simulink model "CF010A_GmTqArbn"  (R2013b)
settings: Solver=FixedStepDiscrete  SolverMode=SingleTasking  StartTime=0.0  StopTime=1  FixedStep=0.002  RelTol=1e-3
values from neighbouring files (symbols this model uses):
  ARCHGLBPRM_2MILLISEC_SEC_F32 = DataDict.Constant    [CF010A_GmTqArbn_DataDict.m]
  ESCTQCMDOVRLLIM_HWNWTMTR_F32 = DataDict.Constant    [CF010A_GmTqArbn_DataDict.m]
  FINALSLEWLWRLIM_HWNWTMTRPERSEC_F32 = DataDict.Constant    [CF010A_GmTqArbn_DataDict.m]
  GmTqArbnApaAssiScaEna = DataDict.Calibration    [CF010A_GmTqArbn_DataDict.m]
  GmTqArbnApaDampgScaEna = DataDict.Calibration    [CF010A_GmTqArbn_DataDict.m]
  GmTqArbnApaEnaRate = DataDict.Calibration    [CF010A_GmTqArbn_DataDict.m]
  GmTqArbnApaRtnScaEna = DataDict.Calibration    [CF010A_GmTqArbn_DataDict.m]
  GmTqArbnEscMaxTq = DataDict.Calibration    [CF010A_GmTqArbn_DataDict.m]
  GmTqArbnLkaOutpOvrlUpprLim = DataDict.Calibration    [CF010A_GmTqArbn_DataDict.m]
  GmTqArbnLkaSlewEna = DataDict.Calibration    [CF010A_GmTqArbn_DataDict.m]
  HWTQCMDOVRLLIM_HWNWTMTR_F32 = DataDict.Constant    [CF010A_GmTqArbn_DataDict.m]
  LKACMDHILIM_HWNWTMTR_F32 = DataDict.Constant    [CF010A_GmTqArbn_DataDict.m]
  LKAOUTPOVRLLIM_MOTNWTMTR_F32 = DataDict.Constant    [CF010A_GmTqArbn_DataDict.m]
  LKATQCMDOVRLLIM_HWNWTMTR_F32 = DataDict.Constant    [CF010A_GmTqArbn_DataDict.m]
  MOTTQCMDOVRLLIM_MOTNWTMTR_F32 = DataDict.Constant    [CF010A_GmTqArbn_DataDict.m]
  OUTPCMDHILIM_ULS_F32 = DataDict.Constant    [CF010A_GmTqArbn_DataDict.m]
  OUTPCMDLOWRLIM_ULS_F32 = DataDict.Constant    [CF010A_GmTqArbn_DataDict.m]
  POSNSERVOSMOOTHMINLWRLIM_ULSPERSEC_F32 = DataDict.Constant    [CF010A_GmTqArbn_DataDict.m]
  VELDPTTQOVRLMTRCOFFS_HWNWTMTRPERSEC_F32 = DataDict.Constant    [CF010A_GmTqArbn_DataDict.m]
  VELDPTTQOVRLMTRCTQPERVEHSPD_HWNWTMTRPERSECPERKPH_F32 = DataDict.Constant    [CF010A_GmTqArbn_DataDict.m]
undefined symbols (not defined in the file or in its folder): GmTqArbnEscSt1, GmTqArbnLkaSt1
libraries: NxtrLim x12, simulink x10, NexteerUtilities x8, FixdToFloat x4, NxtrAbslt x3, Fil x2, FloatToFixd x2, BilnrIntrpnMplX x1, NxtrSign x1
(part 2 of 5)

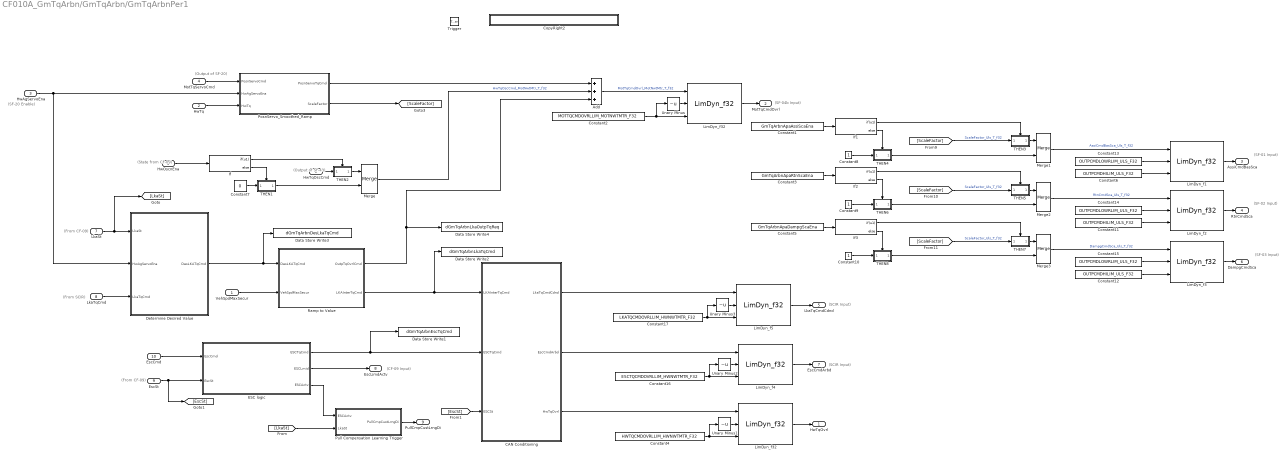
== system CF010A_GmTqArbn/GmTqArbn/GmTqArbnPer1 ==
  note: (SCIR Input)
  note: (SCIR Input)
  note: (SF-03 Input)
  note: (SF-02 Input)
  note: (SF-01 Input)
  note: (SF-04b Input)
  note: (From SCIR)
  note: (From CF-09)
  note: (From CF-09)
  note: (CF-09 Input)
  note: (State from CF-09)
  note: (Output of SF-20)
  note: (SF-20 Enable)
  note: (Output of SF-43)
  VehSpdMaxSecur : Inport  RequirementInfo="{'linktype_rmi_doors' '0000c6e3 (/E-STEER Core/SubSystem Specifications/Customer Functions - EA4/GM/CF010A GM Torque Arbitrator)' '#CF010A_70' 'true' 'REQ:  CF010A_70' '' } %GIDa_f4c84d2e_6e13_4e89_82af_2121b43b1957"
  HwTq : Inport  RequirementInfo="{'linktype_rmi_doors' '0000c6e3 (/E-STEER Core/SubSystem Specifications/Customer Functions - EA4/GM/CF010A GM Torque Arbitrator)' '#CF010A_85' 'true' 'REQ:  CF010A_85' '' } %GIDa_d6d22aaa_d1eb_4354_898c_ba1a58eb138e"  Port=2
  HwAgServoEna : Inport  RequirementInfo="{'linktype_rmi_doors' '0000c6e3 (/E-STEER Core/SubSystem Specifications/Customer Functions - EA4/GM/CF010A GM Torque Arbitrator)' '#CF010A_80' 'true' 'REQ:  CF010A_80' '' ; 'linktype_rmi_doors' '0000c6e3 (/E-STEER Core/SubSystem Specifications/Customer Functions - EA4/GM/CF010A GM Torque Arbitrator)' '#CF010A_83' 'true' 'REQ:  CF010A_83' '' } %GIDa_dd615698_5ebc_469d_8d8d_60e8f236569b"  Port=3
  MotTqServoCmd : Inport  RequirementInfo="{'linktype_rmi_doors' '0000c6e3 (/E-STEER Core/SubSystem Specifications/Customer Functions - EA4/GM/CF010A GM Torque Arbitrator)' '#CF010A_83' 'true' 'REQ:  CF010A_83' '' } %GIDa_295523ce_1dfa_49ab_99cd_a0ea61859de1"  Port=4
  HwOscnEna : Inport  RequirementInfo="{'linktype_rmi_doors' '0000c6e3 (/E-STEER Core/SubSystem Specifications/Customer Functions - EA4/GM/CF010A GM Torque Arbitrator)' '#CF010A_92' 'true' 'REQ:  CF010A_92' '' } %GIDa_b2719311_0b4e_4871_a538_fb1e84a46c67"  Port=5
  HwTqOscCmd : Inport  RequirementInfo="{'linktype_rmi_doors' '0000c6e3 (/E-STEER Core/SubSystem Specifications/Customer Functions - EA4/GM/CF010A GM Torque Arbitrator)' '#CF010A_92' 'true' 'REQ:  CF010A_92' '' } %GIDa_6249b7e4_10fd_4f02_9985_7c0af31baa3d"  Port=6
  LkaSt : Inport  RequirementInfo="{'linktype_rmi_doors' '0000c6e3 (/E-STEER Core/SubSystem Specifications/Customer Functions - EA4/GM/CF010A GM Torque Arbitrator)' '#CF010A_80' 'true' 'REQ:  CF010A_80' '' } %GIDa_90a914dc_c58b_4931_9ec5_c9ec067d425f"  Port=7
  LkaTqCmd : Inport  RequirementInfo="{'linktype_rmi_doors' '0000c6e3 (/E-STEER Core/SubSystem Specifications/Customer Functions - EA4/GM/CF010A GM Torque Arbitrator)' '#CF010A_74' 'true' 'REQ:  CF010A_74' '' } %GIDa_722124bc_7b78_4c03_ae18_255a0a801a18"  Port=8
  EscSt : Inport  RequirementInfo="{'linktype_rmi_doors' '0000c6e3 (/E-STEER Core/SubSystem Specifications/Customer Functions - EA4/GM/CF010A GM Torque Arbitrator)' '#CF010A_104' 'true' 'REQ:  CF010A_104' '' } %GIDa_13f2a128_ed32_48fc_8b3d_535a4820d393"  Port=9
  EscCmd : Inport  RequirementInfo="{'linktype_rmi_doors' '0000c6e3 (/E-STEER Core/SubSystem Specifications/Customer Functions - EA4/GM/CF010A GM Torque Arbitrator)' '#CF010A_77' 'true' 'REQ:  CF010A_77' '' } %GIDa_7431ce68_be09_4736_9e35_35e171474972"  Port=10
  Trigger : TriggerPort  TriggerType=function-call  PortDimensions=1
  Add : Sum  RequirementInfo="{'linktype_rmi_doors' '0000c6e3 (/E-STEER Core/SubSystem Specifications/Customer Functions - EA4/GM/CF010A GM Torque Arbitrator)' '#CF010A_92' 'true' 'REQ:  CF010A_92' '' } %GIDa_443b16ea_0ac5_48aa_b912_06bc53538838"  Inputs=+++
  CAN Conditioning : Subsystem  RequirementInfo="{'linktype_rmi_doors' '0000c6e3 (/E-STEER Core/SubSystem Specifications/Customer Functions - EA4/GM/CF010A GM Torque Arbitrator)' '#CF010A_104' 'true' 'REQ:  CF010A_104' '' ; 'linktype_rmi_doors' '0000c6e3 (/E-STEER Core/SubSystem Specifications/Customer Functions - EA4/GM/CF010A GM Torque Arbitrator)' '#CF010A_79' 'true' 'REQ:  CF010A_79' '' ; 'linktype_rmi_doors' '0000c6e3 (/E-STEER Core/SubSystem Specifications/Customer Functions - EA4/GM/CF010A GM Torque Arbitrator)' '#CF010A_78' 'true' 'REQ:  CF010A_78' '' } %GIDa_54493947_dab7_42c1_b8cc_537cf55edd31"
  Constant1 : Constant  RequirementInfo="{'linktype_rmi_doors' '0000c6e3 (/E-STEER Core/SubSystem Specifications/Customer Functions - EA4/GM/CF010A GM Torque Arbitrator)' '#CF010A_88' 'true' 'REQ:  CF010A_88' '' ; 'linktype_rmi_doors' '0000c6e3 (/E-STEER Core/SubSystem Specifications/Customer Functions - EA4/GM/CF010A GM Torque Arbitrator)' '#CF010A_106' 'true' 'REQ:  CF010A_106' '' } %GIDa_9f4ec867_9728_433f_836c_81d9cdbc89fe"  Value=GmTqArbnApaAssiScaEna
  Constant10 : Constant  RequirementInfo="{'linktype_rmi_doors' '0000c6e3 (/E-STEER Core/SubSystem Specifications/Customer Functions - EA4/GM/CF010A GM Torque Arbitrator)' '#CF010A_106' 'true' 'REQ:  CF010A_106' '' } %GIDa_cd5bc8e1_bd88_45a9_b733_738f1e509e8d"  OutDataTypeStr=single
  Constant11 : Constant  RequirementInfo="{'linktype_rmi_doors' '0000c6e3 (/E-STEER Core/SubSystem Specifications/Customer Functions - EA4/GM/CF010A GM Torque Arbitrator)' '#CF010A_106' 'true' 'REQ:  CF010A_106' '' ; 'linktype_rmi_doors' '0000c6e3 (/E-STEER Core/SubSystem Specifications/Customer Functions - EA4/GM/CF010A GM Torque Arbitrator)' '#CF010A_89' 'true' 'REQ:  CF010A_89' '' ; 'linktype_rmi_doors' '0000c6e3 (/E-STEER Core/SubSystem Specifications/Customer Functions - EA4/GM/CF010A GM Torque Arbitrator)' '#CF010A_98' 'true' 'REQ:  CF010A_98' '' } %GIDa_dee9bf49_23cf_4c3c_9f1e_9ce02392b1a6"  Value=OUTPCMDHILIM_ULS_F32
  Constant12 : Constant  RequirementInfo="{'linktype_rmi_doors' '0000c6e3 (/E-STEER Core/SubSystem Specifications/Customer Functions - EA4/GM/CF010A GM Torque Arbitrator)' '#CF010A_106' 'true' 'REQ:  CF010A_106' '' ; 'linktype_rmi_doors' '0000c6e3 (/E-STEER Core/SubSystem Specifications/Customer Functions - EA4/GM/CF010A GM Torque Arbitrator)' '#CF010A_90' 'true' 'REQ:  CF010A_90' '' ; 'linktype_rmi_doors' '0000c6e3 (/E-STEER Core/SubSystem Specifications/Customer Functions - EA4/GM/CF010A GM Torque Arbitrator)' '#CF010A_99' 'true' 'REQ:  CF010A_99' '' } %GIDa_d68e6ec5_a513_42ff_b0f0_5ecf55882eb9"  Value=OUTPCMDHILIM_ULS_F32
  Constant13 : Constant  RequirementInfo="{'linktype_rmi_doors' '0000c6e3 (/E-STEER Core/SubSystem Specifications/Customer Functions - EA4/GM/CF010A GM Torque Arbitrator)' '#CF010A_88' 'true' 'REQ:  CF010A_88' '' ; 'linktype_rmi_doors' '0000c6e3 (/E-STEER Core/SubSystem Specifications/Customer Functions - EA4/GM/CF010A GM Torque Arbitrator)' '#CF010A_106' 'true' 'REQ:  CF010A_106' '' ; 'linktype_rmi_doors' '0000c6e3 (/E-STEER Core/SubSystem Specifications/Customer Functions - EA4/GM/CF010A GM Torque Arbitrator)' '#CF010A_97' 'true' 'REQ:  CF010A_97' '' } %GIDa_33202896_20d6_4cbc_8518_c46cf7c50787"  Value=OUTPCMDLOWRLIM_ULS_F32
  Constant14 : Constant  RequirementInfo="{'linktype_rmi_doors' '0000c6e3 (/E-STEER Core/SubSystem Specifications/Customer Functions - EA4/GM/CF010A GM Torque Arbitrator)' '#CF010A_106' 'true' 'REQ:  CF010A_106' '' ; 'linktype_rmi_doors' '0000c6e3 (/E-STEER Core/SubSystem Specifications/Customer Functions - EA4/GM/CF010A GM Torque Arbitrator)' '#CF010A_89' 'true' 'REQ:  CF010A_89' '' ; 'linktype_rmi_doors' '0000c6e3 (/E-STEER Core/SubSystem Specifications/Customer Functions - EA4/GM/CF010A GM Torque Arbitrator)' '#CF010A_98' 'true' 'REQ:  CF010A_98' '' } %GIDa_34d37225_e1c2_4150_9259_f5896fb1810b"  Value=OUTPCMDLOWRLIM_ULS_F32
  Constant15 : Constant  RequirementInfo="{'linktype_rmi_doors' '0000c6e3 (/E-STEER Core/SubSystem Specifications/Customer Functions - EA4/GM/CF010A GM Torque Arbitrator)' '#CF010A_106' 'true' 'REQ:  CF010A_106' '' ; 'linktype_rmi_doors' '0000c6e3 (/E-STEER Core/SubSystem Specifications/Customer Functions - EA4/GM/CF010A GM Torque Arbitrator)' '#CF010A_90' 'true' 'REQ:  CF010A_90' '' ; 'linktype_rmi_doors' '0000c6e3 (/E-STEER Core/SubSystem Specifications/Customer Functions - EA4/GM/CF010A GM Torque Arbitrator)' '#CF010A_99' 'true' 'REQ:  CF010A_99' '' } %GIDa_2847f4f8_71a1_405c_87e9_535e82b08a02"  Value=OUTPCMDLOWRLIM_ULS_F32
  Constant16 : Constant  RequirementInfo="{'linktype_rmi_doors' '0000c6e3 (/E-STEER Core/SubSystem Specifications/Customer Functions - EA4/GM/CF010A GM Torque Arbitrator)' '#CF010A_101' 'true' 'REQ:  CF010A_101' '' } %GIDa_704523a7_f0a7_489d_a6ba_a0f7a4852686"  Value=ESCTQCMDOVRLLIM_HWNWTMTR_F32
  Constant17 : Constant  RequirementInfo="{'linktype_rmi_doors' '0000c6e3 (/E-STEER Core/SubSystem Specifications/Customer Functions - EA4/GM/CF010A GM Torque Arbitrator)' '#CF010A_100' 'true' 'REQ:  CF010A_100' '' } %GIDa_2185d7e9_3cba_4308_9a79_783d0e6bbd8b"  Value=LKATQCMDOVRLLIM_HWNWTMTR_F32
  Constant2 : Constant  RequirementInfo="{'linktype_rmi_doors' '0000c6e3 (/E-STEER Core/SubSystem Specifications/Customer Functions - EA4/GM/CF010A GM Torque Arbitrator)' '#CF010A_96' 'true' 'REQ:  CF010A_96' '' } %GIDa_d7f6cff0_b6f2_4ab1_81e2_377ece9f30f8"  Value=MOTTQCMDOVRLLIM_MOTNWTMTR_F32
  Constant3 : Constant  RequirementInfo="{'linktype_rmi_doors' '0000c6e3 (/E-STEER Core/SubSystem Specifications/Customer Functions - EA4/GM/CF010A GM Torque Arbitrator)' '#CF010A_106' 'true' 'REQ:  CF010A_106' '' ; 'linktype_rmi_doors' '0000c6e3 (/E-STEER Core/SubSystem Specifications/Customer Functions - EA4/GM/CF010A GM Torque Arbitrator)' '#CF010A_89' 'true' 'REQ:  CF010A_89' '' } %GIDa_625bdc05_e7d4_43d8_94ec_df5b2f7b5c7f"  Value=GmTqArbnApaRtnScaEna
  Constant4 : Constant  RequirementInfo="{'linktype_rmi_doors' '0000c6e3 (/E-STEER Core/SubSystem Specifications/Customer Functions - EA4/GM/CF010A GM Torque Arbitrator)' '#CF010A_95' 'true' 'REQ:  CF010A_95' '' } %GIDa_07658544_e9ea_4ad2_9c14_704fbb84d33d"  Value=HWTQCMDOVRLLIM_HWNWTMTR_F32
  Constant5 : Constant  RequirementInfo="{'linktype_rmi_doors' '0000c6e3 (/E-STEER Core/SubSystem Specifications/Customer Functions - EA4/GM/CF010A GM Torque Arbitrator)' '#CF010A_106' 'true' 'REQ:  CF010A_106' '' ; 'linktype_rmi_doors' '0000c6e3 (/E-STEER Core/SubSystem Specifications/Customer Functions - EA4/GM/CF010A GM Torque Arbitrator)' '#CF010A_90' 'true' 'REQ:  CF010A_90' '' } %GIDa_45c6d50e_c09d_41c1_9d1e_60f8e7427108"  Value=GmTqArbnApaDampgScaEna
  Constant6 : Constant  RequirementInfo="{'linktype_rmi_doors' '0000c6e3 (/E-STEER Core/SubSystem Specifications/Customer Functions - EA4/GM/CF010A GM Torque Arbitrator)' '#CF010A_88' 'true' 'REQ:  CF010A_88' '' ; 'linktype_rmi_doors' '0000c6e3 (/E-STEER Core/SubSystem Specifications/Customer Functions - EA4/GM/CF010A GM Torque Arbitrator)' '#CF010A_106' 'true' 'REQ:  CF010A_106' '' ; 'linktype_rmi_doors' '0000c6e3 (/E-STEER Core/SubSystem Specifications/Customer Functions - EA4/GM/CF010A GM Torque Arbitrator)' '#CF010A_97' 'true' 'REQ:  CF010A_97' '' } %GIDa_595695da_b2e3_4204_bebc_4d3c88f333a5"  Value=OUTPCMDHILIM_ULS_F32
  Constant7 : Constant  RequirementInfo="{'linktype_rmi_doors' '0000c6e3 (/E-STEER Core/SubSystem Specifications/Customer Functions - EA4/GM/CF010A GM Torque Arbitrator)' '#CF010A_92' 'true' 'REQ:  CF010A_92' '' } %GIDa_5c10319f_4840_4870_a347_6843f256d6f6"  Value=0  OutDataTypeStr=single
  Constant8 : Constant  RequirementInfo="{'linktype_rmi_doors' '0000c6e3 (/E-STEER Core/SubSystem Specifications/Customer Functions - EA4/GM/CF010A GM Torque Arbitrator)' '#CF010A_106' 'true' 'REQ:  CF010A_106' '' } %GIDa_88ffd323_0361_49c8_982c_bfa04abb0131"  OutDataTypeStr=single
  Constant9 : Constant  RequirementInfo="{'linktype_rmi_doors' '0000c6e3 (/E-STEER Core/SubSystem Specifications/Customer Functions - EA4/GM/CF010A GM Torque Arbitrator)' '#CF010A_106' 'true' 'REQ:  CF010A_106' '' } %GIDa_0fc4b1f9_c465_47be_a1c4_e4799872c48e"  OutDataTypeStr=single
  CopyRight2 : Subsystem  Description=|  mask(Copyright Information){none=on}
      | Copyright info block.                                               
      |                                                                     
      | Place copyright information at the top of every subsystem in design.
      mask prompts: none "No parameters"
      mask help: Place copyright information at the top of every subsystem in design.
      mask Display:
      | NxtrConf = 'Nexteer Confidential';
      | 
      | sys = bdroot; %handle for the current model ("system")
      | first = get_param(sys,'Created');
      | first = first(end-3:end);  %year is last four digits
      | 
      | last = get_param(sys,'LastModifiedDate');
      | if isempty(last)
      |     last = datestr(now,'yyyy');
      | else
      |     last = last(end-3:end);
      | end
      | 
      | if strcmp(first,last)
      |     fprintf('%s -- Copyright %s Nexteer',NxtrConf,first)
      | else
      |     fprintf('%s -- %s%s- %s Nexteer',NxtrConf,char(169),first,last)
      | end
  Data Store Write1 : DataStoreWrite  DataStoreName=dGmTqArbnEscTqCmd
  Data Store Write2 : DataStoreWrite  DataStoreName=dGmTqArbnLkaTqCmd
  Data Store Write3 : DataStoreWrite  DataStoreName=dGmTqArbnDesLkaTqCmd
  Data Store Write4 : DataStoreWrite  DataStoreName=dGmTqArbnLkaOutpTqReq
  Determine Desired Value : Subsystem  RequirementInfo={} %GIDa_93b3e7d5_080f_4803_8517_c119903720fd
  ESC logic : Subsystem
  If : If  RequirementInfo="{'linktype_rmi_doors' '0000c6e3 (/E-STEER Core/SubSystem Specifications/Customer Functions - EA4/GM/CF010A GM Torque Arbitrator)' '#CF010A_92' 'true' 'REQ:  CF010A_92' '' } %GIDa_6e19b322_c53d_4317_8726_22c74644b724"  IfExpression=u1
  If1 : If  RequirementInfo="{'linktype_rmi_doors' '0000c6e3 (/E-STEER Core/SubSystem Specifications/Customer Functions - EA4/GM/CF010A GM Torque Arbitrator)' '#CF010A_88' 'true' 'REQ:  CF010A_88' '' ; 'linktype_rmi_doors' '0000c6e3 (/E-STEER Core/SubSystem Specifications/Customer Functions - EA4/GM/CF010A GM Torque Arbitrator)' '#CF010A_106' 'true' 'REQ:  CF010A_106' '' } %GIDa_3e0680a5_b2e6_45d9_b4ba_d1ec68cc74dc"  IfExpression=u1
  If2 : If  RequirementInfo="{'linktype_rmi_doors' '0000c6e3 (/E-STEER Core/SubSystem Specifications/Customer Functions - EA4/GM/CF010A GM Torque Arbitrator)' '#CF010A_106' 'true' 'REQ:  CF010A_106' '' ; 'linktype_rmi_doors' '0000c6e3 (/E-STEER Core/SubSystem Specifications/Customer Functions - EA4/GM/CF010A GM Torque Arbitrator)' '#CF010A_89' 'true' 'REQ:  CF010A_89' '' } %GIDa_1656b378_739f_4f97_a3c7_2e960e9b6287"  IfExpression=u1
  If3 : If  RequirementInfo="{'linktype_rmi_doors' '0000c6e3 (/E-STEER Core/SubSystem Specifications/Customer Functions - EA4/GM/CF010A GM Torque Arbitrator)' '#CF010A_106' 'true' 'REQ:  CF010A_106' '' ; 'linktype_rmi_doors' '0000c6e3 (/E-STEER Core/SubSystem Specifications/Customer Functions - EA4/GM/CF010A GM Torque Arbitrator)' '#CF010A_90' 'true' 'REQ:  CF010A_90' '' } %GIDa_13fb500e_8bdd_499f_8d05_46c9f37ebc1e"  IfExpression=u1
  LimDyn_f1 : NxtrLim/LimDyn_f32  RequirementInfo="{'linktype_rmi_doors' '0000c6e3 (/E-STEER Core/SubSystem Specifications/Customer Functions - EA4/GM/CF010A GM Torque Arbitrator)' '#CF010A_88' 'true' 'REQ:  CF010A_88' '' ; 'linktype_rmi_doors' '0000c6e3 (/E-STEER Core/SubSystem Specifications/Customer Functions - EA4/GM/CF010A GM Torque Arbitrator)' '#CF010A_106' 'true' 'REQ:  CF010A_106' '' ; 'linktype_rmi_doors' '0000c6e3 (/E-STEER Core/SubSystem Specifications/Customer Functions - EA4/GM/CF010A GM Torque Arbitrator)' '#CF010A_97' 'true' 'REQ:  CF010A_97' '' } %GIDa_eb308def_f76b_4d03_bc15_1f722664d519"
  LimDyn_f2 : NxtrLim/LimDyn_f32  RequirementInfo="{'linktype_rmi_doors' '0000c6e3 (/E-STEER Core/SubSystem Specifications/Customer Functions - EA4/GM/CF010A GM Torque Arbitrator)' '#CF010A_106' 'true' 'REQ:  CF010A_106' '' ; 'linktype_rmi_doors' '0000c6e3 (/E-STEER Core/SubSystem Specifications/Customer Functions - EA4/GM/CF010A GM Torque Arbitrator)' '#CF010A_89' 'true' 'REQ:  CF010A_89' '' ; 'linktype_rmi_doors' '0000c6e3 (/E-STEER Core/SubSystem Specifications/Customer Functions - EA4/GM/CF010A GM Torque Arbitrator)' '#CF010A_98' 'true' 'REQ:  CF010A_98' '' } %GIDa_1aa4b260_59c5_461f_9c0a_7bc3cdfd86c1"
  LimDyn_f3 : NxtrLim/LimDyn_f32  RequirementInfo="{'linktype_rmi_doors' '0000c6e3 (/E-STEER Core/SubSystem Specifications/Customer Functions - EA4/GM/CF010A GM Torque Arbitrator)' '#CF010A_106' 'true' 'REQ:  CF010A_106' '' ; 'linktype_rmi_doors' '0000c6e3 (/E-STEER Core/SubSystem Specifications/Customer Functions - EA4/GM/CF010A GM Torque Arbitrator)' '#CF010A_90' 'true' 'REQ:  CF010A_90' '' ; 'linktype_rmi_doors' '0000c6e3 (/E-STEER Core/SubSystem Specifications/Customer Functions - EA4/GM/CF010A GM Torque Arbitrator)' '#CF010A_99' 'true' 'REQ:  CF010A_99' '' } %GIDa_4b0d240a_aaa3_4679_a6ee_cace697a3954"
  LimDyn_f32 : NxtrLim/LimDyn_f32  RequirementInfo="{'linktype_rmi_doors' '0000c6e3 (/E-STEER Core/SubSystem Specifications/Customer Functions - EA4/GM/CF010A GM Torque Arbitrator)' '#CF010A_95' 'true' 'REQ:  CF010A_95' '' } %GIDa_40620354_0f4e_4aa0_8156_4e529ce3c86d"
  "LimDyn_f32 " : NxtrLim/LimDyn_f32  RequirementInfo="{'linktype_rmi_doors' '0000c6e3 (/E-STEER Core/SubSystem Specifications/Customer Functions - EA4/GM/CF010A GM Torque Arbitrator)' '#CF010A_96' 'true' 'REQ:  CF010A_96' '' } %GIDa_1898a333_229b_4680_8fe2_3a06d3151cf7"
  LimDyn_f4 : NxtrLim/LimDyn_f32  RequirementInfo="{'linktype_rmi_doors' '0000c6e3 (/E-STEER Core/SubSystem Specifications/Customer Functions - EA4/GM/CF010A GM Torque Arbitrator)' '#CF010A_101' 'true' 'REQ:  CF010A_101' '' } %GIDa_17cbc088_da8d_4e32_82d9_cddfa289c580"
  LimDyn_f5 : NxtrLim/LimDyn_f32  RequirementInfo="{'linktype_rmi_doors' '0000c6e3 (/E-STEER Core/SubSystem Specifications/Customer Functions - EA4/GM/CF010A GM Torque Arbitrator)' '#CF010A_100' 'true' 'REQ:  CF010A_100' '' } %GIDa_c57b82a9_e331_4a03_9062_9a6e5a59a2ed"
  Merge : Merge  RequirementInfo="{'linktype_rmi_doors' '0000c6e3 (/E-STEER Core/SubSystem Specifications/Customer Functions - EA4/GM/CF010A GM Torque Arbitrator)' '#CF010A_92' 'true' 'REQ:  CF010A_92' '' } %GIDa_77d22198_c62c_4175_bf35_c7728d9b6201"
  Merge1 : Merge  RequirementInfo="{'linktype_rmi_doors' '0000c6e3 (/E-STEER Core/SubSystem Specifications/Customer Functions - EA4/GM/CF010A GM Torque Arbitrator)' '#CF010A_88' 'true' 'REQ:  CF010A_88' '' ; 'linktype_rmi_doors' '0000c6e3 (/E-STEER Core/SubSystem Specifications/Customer Functions - EA4/GM/CF010A GM Torque Arbitrator)' '#CF010A_106' 'true' 'REQ:  CF010A_106' '' } %GIDa_1934bf47_1b49_4b5a_9848_768905c53dba"
  Merge2 : Merge  RequirementInfo="{'linktype_rmi_doors' '0000c6e3 (/E-STEER Core/SubSystem Specifications/Customer Functions - EA4/GM/CF010A GM Torque Arbitrator)' '#CF010A_106' 'true' 'REQ:  CF010A_106' '' ; 'linktype_rmi_doors' '0000c6e3 (/E-STEER Core/SubSystem Specifications/Customer Functions - EA4/GM/CF010A GM Torque Arbitrator)' '#CF010A_89' 'true' 'REQ:  CF010A_89' '' } %GIDa_9e6b0280_be22_44d1_a6f0_1053f8e0b771"
  Merge3 : Merge  RequirementInfo="{'linktype_rmi_doors' '0000c6e3 (/E-STEER Core/SubSystem Specifications/Customer Functions - EA4/GM/CF010A GM Torque Arbitrator)' '#CF010A_106' 'true' 'REQ:  CF010A_106' '' ; 'linktype_rmi_doors' '0000c6e3 (/E-STEER Core/SubSystem Specifications/Customer Functions - EA4/GM/CF010A GM Torque Arbitrator)' '#CF010A_90' 'true' 'REQ:  CF010A_90' '' } %GIDa_f03aa417_b741_49cc_b9a6_95614de85211"
  PosnServo_Smoothed_Ramp : Subsystem
  Pull Compensation Learning Trigger : Subsystem  RequirementInfo="{'linktype_rmi_doors' '0000c6e3 (/E-STEER Core/SubSystem Specifications/Customer Functions - EA4/GM/CF010A GM Torque Arbitrator)' '#CF010A_113' 'true' 'REQ:  CF010A_113' '' } %GIDa_af075b18_56f7_4ac0_b6c2_3a4816aa02fc"
  Ramp to Value : Subsystem
  THEN1 : Subsystem  RequirementInfo="{'linktype_rmi_doors' '0000c6e3 (/E-STEER Core/SubSystem Specifications/Customer Functions - EA4/GM/CF010A GM Torque Arbitrator)' '#CF010A_92' 'true' 'REQ:  CF010A_92' '' } %GIDa_b260fa9c_4cdb_4aaa_ae2f_69ac7f8b672c"  TreatAsAtomicUnit=on  mask(pass thru, version Nov 30, 2012){nIn=1}
      mask prompts: nIn "Number of input signals"
      mask help:
      | This block passes its input straight through without modification.
      |
      | Enter the number of signals to pass through (integer 1 to 5).
      mask Callback nIn:
      | thisBlock = gcb;
      | a = get_param(thisBlock,'MaskValues');
      | b = cell2mat(a);
      | c = str2num(b);
      | 
      | if c<1 c=1; end
      | if c>5 c=5; end
      | 
      | for idx=1:c
      |     sIdx = num2str(idx);
      |     oldblock = [thisBlock '/In' sIdx];
      |     if strcmp(get_param(oldblock,'BlockType'),'Ground')
      |          newblock = 'built-in/Inport';
      |         pos = get_param(oldblock,'Position');
      |         orient = get_param(oldblock,'Orientation');
      |         delete_block(oldblock);
      |         add_block(newblock,oldblock,'Position',pos, 'Orientation',orient);
      |     end
      | 
      |     oldblock = [thisBlock '/Out' sIdx];
      |     if strcmp(get_param(oldblock,'BlockType'),'Terminator')
      |         newblock = 'built-in/Outport';
      |         pos = get_param(oldblock,'Position');
      |         orient = get_param(oldblock,'Orientation');
      |         delete_block(oldblock);
      |         add_block(newblock,oldblock,'Position',pos, 'Orientation',orient);
      |     end
      | end
      | 
      | for idx=c+1:5
      |     sIdx = num2str(idx);
      |     oldblock = [thisBlock '/In' sIdx];
      |     if strcmp(get_param(oldblock,'BlockType'),'Inport')
      |         newblock = 'built-in/Ground';
      |         pos = get_param(oldblock,'Position');
      |         orient = get_param(oldblock,'Orientation');
      |         delete_block(oldblock);
      |         add_block(newblock,oldblock,'Position',pos, 'Orientation',orient);
      |     end
      | 
      |     oldblock = [thisBlock '/Out' sIdx];
      |     if strcmp(get_param(oldblock,'BlockType'),'Outport')
      |         newblock = 'built-in/Terminator';
      |         pos = get_param(oldblock,'Position');
      |         orient = get_param(oldblock,'Orientation');
      |         delete_block(oldblock);
      |         add_block(newblock,oldblock,'Position',pos, 'Orientation',orient);
      |     end
      | end
      | 
      | 
      | 
      | clear thisBlock oldblock newblock orient pos a b c idx sIdx ;
      mask Display: fprintf('pass\nthru')
  THEN2 : Subsystem  RequirementInfo="{'linktype_rmi_doors' '0000c6e3 (/E-STEER Core/SubSystem Specifications/Customer Functions - EA4/GM/CF010A GM Torque Arbitrator)' '#CF010A_92' 'true' 'REQ:  CF010A_92' '' } %GIDa_5bde3786_d9f4_4ae5_940c_87d032de86d5"  TreatAsAtomicUnit=on  mask(pass thru, version Nov 30, 2012){nIn=1}
      mask prompts: nIn "Number of input signals"
      mask help:
      | This block passes its input straight through without modification.
      |
      | Enter the number of signals to pass through (integer 1 to 5).
      mask Callback nIn:
      | thisBlock = gcb;
      | a = get_param(thisBlock,'MaskValues');
      | b = cell2mat(a);
      | c = str2num(b);
      | 
      | if c<1 c=1; end
      | if c>5 c=5; end
      | 
      | for idx=1:c
      |     sIdx = num2str(idx);
      |     oldblock = [thisBlock '/In' sIdx];
      |     if strcmp(get_param(oldblock,'BlockType'),'Ground')
      |          newblock = 'built-in/Inport';
      |         pos = get_param(oldblock,'Position');
      |         orient = get_param(oldblock,'Orientation');
      |         delete_block(oldblock);
      |         add_block(newblock,oldblock,'Position',pos, 'Orientation',orient);
      |     end
      | 
      |     oldblock = [thisBlock '/Out' sIdx];
      |     if strcmp(get_param(oldblock,'BlockType'),'Terminator')
      |         newblock = 'built-in/Outport';
      |         pos = get_param(oldblock,'Position');
      |         orient = get_param(oldblock,'Orientation');
      |         delete_block(oldblock);
      |         add_block(newblock,oldblock,'Position',pos, 'Orientation',orient);
      |     end
      | end
      | 
      | for idx=c+1:5
      |     sIdx = num2str(idx);
      |     oldblock = [thisBlock '/In' sIdx];
      |     if strcmp(get_param(oldblock,'BlockType'),'Inport')
      |         newblock = 'built-in/Ground';
      |         pos = get_param(oldblock,'Position');
      |         orient = get_param(oldblock,'Orientation');
      |         delete_block(oldblock);
      |         add_block(newblock,oldblock,'Position',pos, 'Orientation',orient);
      |     end
      | 
      |     oldblock = [thisBlock '/Out' sIdx];
      |     if strcmp(get_param(oldblock,'BlockType'),'Outport')
      |         newblock = 'built-in/Terminator';
      |         pos = get_param(oldblock,'Position');
      |         orient = get_param(oldblock,'Orientation');
      |         delete_block(oldblock);
      |         add_block(newblock,oldblock,'Position',pos, 'Orientation',orient);
      |     end
      | end
      | 
      | 
      | 
      | clear thisBlock oldblock newblock orient pos a b c idx sIdx ;
      mask Display: fprintf('pass\nthru')
  THEN3 : Subsystem  RequirementInfo="{'linktype_rmi_doors' '0000c6e3 (/E-STEER Core/SubSystem Specifications/Customer Functions - EA4/GM/CF010A GM Torque Arbitrator)' '#CF010A_88' 'true' 'REQ:  CF010A_88' '' } %GIDa_d758718b_0144_4eac_9881_31401cf36d2a"  TreatAsAtomicUnit=on  mask(pass thru, version Nov 30, 2012){nIn=1}
      mask prompts: nIn "Number of input signals"
      mask help:
      | This block passes its input straight through without modification.
      |
      | Enter the number of signals to pass through (integer 1 to 5).
      mask Callback nIn:
      | thisBlock = gcb;
      | a = get_param(thisBlock,'MaskValues');
      | b = cell2mat(a);
      | c = str2num(b);
      | 
      | if c<1 c=1; end
      | if c>5 c=5; end
      | 
      | for idx=1:c
      |     sIdx = num2str(idx);
      |     oldblock = [thisBlock '/In' sIdx];
      |     if strcmp(get_param(oldblock,'BlockType'),'Ground')
      |          newblock = 'built-in/Inport';
      |         pos = get_param(oldblock,'Position');
      |         orient = get_param(oldblock,'Orientation');
      |         delete_block(oldblock);
      |         add_block(newblock,oldblock,'Position',pos, 'Orientation',orient);
      |     end
      | 
      |     oldblock = [thisBlock '/Out' sIdx];
      |     if strcmp(get_param(oldblock,'BlockType'),'Terminator')
      |         newblock = 'built-in/Outport';
      |         pos = get_param(oldblock,'Position');
      |         orient = get_param(oldblock,'Orientation');
      |         delete_block(oldblock);
      |         add_block(newblock,oldblock,'Position',pos, 'Orientation',orient);
      |     end
      | end
      | 
      | for idx=c+1:5
      |     sIdx = num2str(idx);
      |     oldblock = [thisBlock '/In' sIdx];
      |     if strcmp(get_param(oldblock,'BlockType'),'Inport')
      |         newblock = 'built-in/Ground';
      |         pos = get_param(oldblock,'Position');
      |         orient = get_param(oldblock,'Orientation');
      |         delete_block(oldblock);
      |         add_block(newblock,oldblock,'Position',pos, 'Orientation',orient);
      |     end
      | 
      |     oldblock = [thisBlock '/Out' sIdx];
      |     if strcmp(get_param(oldblock,'BlockType'),'Outport')
      |         newblock = 'built-in/Terminator';
      |         pos = get_param(oldblock,'Position');
      |         orient = get_param(oldblock,'Orientation');
      |         delete_block(oldblock);
      |         add_block(newblock,oldblock,'Position',pos, 'Orientation',orient);
      |     end
      | end
      | 
      | 
      | 
      | clear thisBlock oldblock newblock orient pos a b c idx sIdx ;
      mask Display: fprintf('pass\nthru')
  THEN4 : Subsystem  RequirementInfo="{'linktype_rmi_doors' '0000c6e3 (/E-STEER Core/SubSystem Specifications/Customer Functions - EA4/GM/CF010A GM Torque Arbitrator)' '#CF010A_106' 'true' 'REQ:  CF010A_106' '' } %GIDa_e1ba3c2d_8fad_48f0_b475_5acb6897d40c"  TreatAsAtomicUnit=on  mask(pass thru, version Nov 30, 2012){nIn=1}
      mask prompts: nIn "Number of input signals"
      mask help:
      | This block passes its input straight through without modification.
      |
      | Enter the number of signals to pass through (integer 1 to 5).
      mask Callback nIn:
      | thisBlock = gcb;
      | a = get_param(thisBlock,'MaskValues');
      | b = cell2mat(a);
      | c = str2num(b);
      | 
      | if c<1 c=1; end
      | if c>5 c=5; end
      | 
      | for idx=1:c
      |     sIdx = num2str(idx);
      |     oldblock = [thisBlock '/In' sIdx];
      |     if strcmp(get_param(oldblock,'BlockType'),'Ground')
      |          newblock = 'built-in/Inport';
      |         pos = get_param(oldblock,'Position');
      |         orient = get_param(oldblock,'Orientation');
      |         delete_block(oldblock);
      |         add_block(newblock,oldblock,'Position',pos, 'Orientation',orient);
      |     end
      | 
      |     oldblock = [thisBlock '/Out' sIdx];
      |     if strcmp(get_param(oldblock,'BlockType'),'Terminator')
      |         newblock = 'built-in/Outport';
      |         pos = get_param(oldblock,'Position');
      |         orient = get_param(oldblock,'Orientation');
      |         delete_block(oldblock);
      |         add_block(newblock,oldblock,'Position',pos, 'Orientation',orient);
      |     end
      | end
      | 
      | for idx=c+1:5
      |     sIdx = num2str(idx);
      |     oldblock = [thisBlock '/In' sIdx];
      |     if strcmp(get_param(oldblock,'BlockType'),'Inport')
      |         newblock = 'built-in/Ground';
      |         pos = get_param(oldblock,'Position');
      |         orient = get_param(oldblock,'Orientation');
      |         delete_block(oldblock);
      |         add_block(newblock,oldblock,'Position',pos, 'Orientation',orient);
      |     end
      | 
      |     oldblock = [thisBlock '/Out' sIdx];
      |     if strcmp(get_param(oldblock,'BlockType'),'Outport')
      |         newblock = 'built-in/Terminator';
      |         pos = get_param(oldblock,'Position');
      |         orient = get_param(oldblock,'Orientation');
      |         delete_block(oldblock);
      |         add_block(newblock,oldblock,'Position',pos, 'Orientation',orient);
      |     end
      | end
      | 
      | 
      | 
      | clear thisBlock oldblock newblock orient pos a b c idx sIdx ;
      mask Display: fprintf('pass\nthru')
  THEN5 : Subsystem  RequirementInfo="{'linktype_rmi_doors' '0000c6e3 (/E-STEER Core/SubSystem Specifications/Customer Functions - EA4/GM/CF010A GM Torque Arbitrator)' '#CF010A_89' 'true' 'REQ:  CF010A_89' '' } %GIDa_fea473c1_093f_4ff2_899d_9142ecda2b9c"  TreatAsAtomicUnit=on  mask(pass thru, version Nov 30, 2012){nIn=1}
      mask prompts: nIn "Number of input signals"
      mask help:
      | This block passes its input straight through without modification.
      |
      | Enter the number of signals to pass through (integer 1 to 5).
      mask Callback nIn:
      | thisBlock = gcb;
      | a = get_param(thisBlock,'MaskValues');
      | b = cell2mat(a);
      | c = str2num(b);
      | 
      | if c<1 c=1; end
      | if c>5 c=5; end
      | 
      | for idx=1:c
      |     sIdx = num2str(idx);
      |     oldblock = [thisBlock '/In' sIdx];
      |     if strcmp(get_param(oldblock,'BlockType'),'Ground')
      |          newblock = 'built-in/Inport';
      |         pos = get_param(oldblock,'Position');
      |         orient = get_param(oldblock,'Orientation');
      |         delete_block(oldblock);
      |         add_block(newblock,oldblock,'Position',pos, 'Orientation',orient);
      |     end
      | 
      |     oldblock = [thisBlock '/Out' sIdx];
      |     if strcmp(get_param(oldblock,'BlockType'),'Terminator')
      |         newblock = 'built-in/Outport';
      |         pos = get_param(oldblock,'Position');
      |         orient = get_param(oldblock,'Orientation');
      |         delete_block(oldblock);
      |         add_block(newblock,oldblock,'Position',pos, 'Orientation',orient);
      |     end
      | end
      | 
      | for idx=c+1:5
      |     sIdx = num2str(idx);
      |     oldblock = [thisBlock '/In' sIdx];
      |     if strcmp(get_param(oldblock,'BlockType'),'Inport')
      |         newblock = 'built-in/Ground';
      |         pos = get_param(oldblock,'Position');
      |         orient = get_param(oldblock,'Orientation');
      |         delete_block(oldblock);
      |         add_block(newblock,oldblock,'Position',pos, 'Orientation',orient);
      |     end
      | 
      |     oldblock = [thisBlock '/Out' sIdx];
      |     if strcmp(get_param(oldblock,'BlockType'),'Outport')
      |         newblock = 'built-in/Terminator';
      |         pos = get_param(oldblock,'Position');
      |         orient = get_param(oldblock,'Orientation');
      |         delete_block(oldblock);
      |         add_block(newblock,oldblock,'Position',pos, 'Orientation',orient);
      |     end
      | end
      | 
      | 
      | 
      | clear thisBlock oldblock newblock orient pos a b c idx sIdx ;
      mask Display: fprintf('pass\nthru')
  THEN6 : Subsystem  RequirementInfo="{'linktype_rmi_doors' '0000c6e3 (/E-STEER Core/SubSystem Specifications/Customer Functions - EA4/GM/CF010A GM Torque Arbitrator)' '#CF010A_106' 'true' 'REQ:  CF010A_106' '' } %GIDa_0d0ff04e_04bf_43f9_88c4_85e73db6cdf4"  TreatAsAtomicUnit=on  mask(pass thru, version Nov 30, 2012){nIn=1}
      mask prompts: nIn "Number of input signals"
      mask help:
      | This block passes its input straight through without modification.
      |
      | Enter the number of signals to pass through (integer 1 to 5).
      mask Callback nIn:
      | thisBlock = gcb;
      | a = get_param(thisBlock,'MaskValues');
      | b = cell2mat(a);
      | c = str2num(b);
      | 
      | if c<1 c=1; end
      | if c>5 c=5; end
      | 
      | for idx=1:c
      |     sIdx = num2str(idx);
      |     oldblock = [thisBlock '/In' sIdx];
      |     if strcmp(get_param(oldblock,'BlockType'),'Ground')
      |          newblock = 'built-in/Inport';
      |         pos = get_param(oldblock,'Position');
      |         orient = get_param(oldblock,'Orientation');
      |         delete_block(oldblock);
      |         add_block(newblock,oldblock,'Position',pos, 'Orientation',orient);
      |     end
      | 
      |     oldblock = [thisBlock '/Out' sIdx];
      |     if strcmp(get_param(oldblock,'BlockType'),'Terminator')
      |         newblock = 'built-in/Outport';
      |         pos = get_param(oldblock,'Position');
      |         orient = get_param(oldblock,'Orientation');
      |         delete_block(oldblock);
      |         add_block(newblock,oldblock,'Position',pos, 'Orientation',orient);
      |     end
      | end
      | 
      | for idx=c+1:5
      |     sIdx = num2str(idx);
      |     oldblock = [thisBlock '/In' sIdx];
      |     if strcmp(get_param(oldblock,'BlockType'),'Inport')
      |         newblock = 'built-in/Ground';
      |         pos = get_param(oldblock,'Position');
      |         orient = get_param(oldblock,'Orientation');
      |         delete_block(oldblock);
      |         add_block(newblock,oldblock,'Position',pos, 'Orientation',orient);
      |     end
      | 
      |     oldblock = [thisBlock '/Out' sIdx];
      |     if strcmp(get_param(oldblock,'BlockType'),'Outport')
      |         newblock = 'built-in/Terminator';
      |         pos = get_param(oldblock,'Position');
      |         orient = get_param(oldblock,'Orientation');
      |         delete_block(oldblock);
      |         add_block(newblock,oldblock,'Position',pos, 'Orientation',orient);
      |     end
      | end
      | 
      | 
      | 
      | clear thisBlock oldblock newblock orient pos a b c idx sIdx ;
      mask Display: fprintf('pass\nthru')
  THEN7 : Subsystem  RequirementInfo="{'linktype_rmi_doors' '0000c6e3 (/E-STEER Core/SubSystem Specifications/Customer Functions - EA4/GM/CF010A GM Torque Arbitrator)' '#CF010A_90' 'true' 'REQ:  CF010A_90' '' } %GIDa_e8415cb2_c251_4c08_9b19_892187c308a4"  TreatAsAtomicUnit=on  mask(pass thru, version Nov 30, 2012){nIn=1}
      mask prompts: nIn "Number of input signals"
      mask help:
      | This block passes its input straight through without modification.
      |
      | Enter the number of signals to pass through (integer 1 to 5).
      mask Callback nIn:
      | thisBlock = gcb;
      | a = get_param(thisBlock,'MaskValues');
      | b = cell2mat(a);
      | c = str2num(b);
      | 
      | if c<1 c=1; end
      | if c>5 c=5; end
      | 
      | for idx=1:c
      |     sIdx = num2str(idx);
      |     oldblock = [thisBlock '/In' sIdx];
      |     if strcmp(get_param(oldblock,'BlockType'),'Ground')
      |          newblock = 'built-in/Inport';
      |         pos = get_param(oldblock,'Position');
      |         orient = get_param(oldblock,'Orientation');
      |         delete_block(oldblock);
      |         add_block(newblock,oldblock,'Position',pos, 'Orientation',orient);
      |     end
      | 
      |     oldblock = [thisBlock '/Out' sIdx];
      |     if strcmp(get_param(oldblock,'BlockType'),'Terminator')
      |         newblock = 'built-in/Outport';
      |         pos = get_param(oldblock,'Position');
      |         orient = get_param(oldblock,'Orientation');
      |         delete_block(oldblock);
      |         add_block(newblock,oldblock,'Position',pos, 'Orientation',orient);
      |     end
      | end
      | 
      | for idx=c+1:5
      |     sIdx = num2str(idx);
      |     oldblock = [thisBlock '/In' sIdx];
      |     if strcmp(get_param(oldblock,'BlockType'),'Inport')
      |         newblock = 'built-in/Ground';
      |         pos = get_param(oldblock,'Position');
      |         orient = get_param(oldblock,'Orientation');
      |         delete_block(oldblock);
      |         add_block(newblock,oldblock,'Position',pos, 'Orientation',orient);
      |     end
      | 
      |     oldblock = [thisBlock '/Out' sIdx];
      |     if strcmp(get_param(oldblock,'BlockType'),'Outport')
      |         newblock = 'built-in/Terminator';
      |         pos = get_param(oldblock,'Position');
      |         orient = get_param(oldblock,'Orientation');
      |         delete_block(oldblock);
      |         add_block(newblock,oldblock,'Position',pos, 'Orientation',orient);
      |     end
      | end
      | 
      | 
      | 
      | clear thisBlock oldblock newblock orient pos a b c idx sIdx ;
      mask Display: fprintf('pass\nthru')
  THEN8 : Subsystem  RequirementInfo="{'linktype_rmi_doors' '0000c6e3 (/E-STEER Core/SubSystem Specifications/Customer Functions - EA4/GM/CF010A GM Torque Arbitrator)' '#CF010A_106' 'true' 'REQ:  CF010A_106' '' } %GIDa_1c38b251_2d22_4757_b5bd_5c35a9eeaa83"  TreatAsAtomicUnit=on  mask(pass thru, version Nov 30, 2012){nIn=1}
      mask prompts: nIn "Number of input signals"
      mask help:
      | This block passes its input straight through without modification.
      |
      | Enter the number of signals to pass through (integer 1 to 5).
      mask Callback nIn:
      | thisBlock = gcb;
      | a = get_param(thisBlock,'MaskValues');
      | b = cell2mat(a);
      | c = str2num(b);
      | 
      | if c<1 c=1; end
      | if c>5 c=5; end
      | 
      | for idx=1:c
      |     sIdx = num2str(idx);
      |     oldblock = [thisBlock '/In' sIdx];
      |     if strcmp(get_param(oldblock,'BlockType'),'Ground')
      |          newblock = 'built-in/Inport';
      |         pos = get_param(oldblock,'Position');
      |         orient = get_param(oldblock,'Orientation');
      |         delete_block(oldblock);
      |         add_block(newblock,oldblock,'Position',pos, 'Orientation',orient);
      |     end
      | 
      |     oldblock = [thisBlock '/Out' sIdx];
      |     if strcmp(get_param(oldblock,'BlockType'),'Terminator')
      |         newblock = 'built-in/Outport';
      |         pos = get_param(oldblock,'Position');
      |         orient = get_param(oldblock,'Orientation');
      |         delete_block(oldblock);
      |         add_block(newblock,oldblock,'Position',pos, 'Orientation',orient);
      |     end
      | end
      | 
      | for idx=c+1:5
      |     sIdx = num2str(idx);
      |     oldblock = [thisBlock '/In' sIdx];
      |     if strcmp(get_param(oldblock,'BlockType'),'Inport')
      |         newblock = 'built-in/Ground';
      |         pos = get_param(oldblock,'Position');
      |         orient = get_param(oldblock,'Orientation');
      |         delete_block(oldblock);
      |         add_block(newblock,oldblock,'Position',pos, 'Orientation',orient);
      |     end
      | 
      |     oldblock = [thisBlock '/Out' sIdx];
      |     if strcmp(get_param(oldblock,'BlockType'),'Outport')
      |         newblock = 'built-in/Terminator';
      |         pos = get_param(oldblock,'Position');
      |         orient = get_param(oldblock,'Orientation');
      |         delete_block(oldblock);
      |         add_block(newblock,oldblock,'Position',pos, 'Orientation',orient);
      |     end
      | end
      | 
      | 
      | 
      | clear thisBlock oldblock newblock orient pos a b c idx sIdx ;
      mask Display: fprintf('pass\nthru')
  Unary Minus : UnaryMinus  RequirementInfo="{'linktype_rmi_doors' '0000c6e3 (/E-STEER Core/SubSystem Specifications/Customer Functions - EA4/GM/CF010A GM Torque Arbitrator)' '#CF010A_96' 'true' 'REQ:  CF010A_96' '' } %GIDa_885a3e5b_5ba9_46b7_8550_7df966f103e8"
  Unary Minus1 : UnaryMinus  RequirementInfo="{'linktype_rmi_doors' '0000c6e3 (/E-STEER Core/SubSystem Specifications/Customer Functions - EA4/GM/CF010A GM Torque Arbitrator)' '#CF010A_95' 'true' 'REQ:  CF010A_95' '' } %GIDa_dfb1c566_b1f8_4658_b404_87a599226837"
  Unary Minus2 : UnaryMinus  RequirementInfo="{'linktype_rmi_doors' '0000c6e3 (/E-STEER Core/SubSystem Specifications/Customer Functions - EA4/GM/CF010A GM Torque Arbitrator)' '#CF010A_101' 'true' 'REQ:  CF010A_101' '' } %GIDa_10f59235_d585_4bb8_a331_4cc5ed205112"
  Unary Minus3 : UnaryMinus  RequirementInfo="{'linktype_rmi_doors' '0000c6e3 (/E-STEER Core/SubSystem Specifications/Customer Functions - EA4/GM/CF010A GM Torque Arbitrator)' '#CF010A_100' 'true' 'REQ:  CF010A_100' '' } %GIDa_94dea463_9d39_4f49_9d48_41451587abc4"
  HwTqOvrl : Outport  RequirementInfo="{'linktype_rmi_doors' '0000c6e3 (/E-STEER Core/SubSystem Specifications/Customer Functions - EA4/GM/CF010A GM Torque Arbitrator)' '#CF010A_104' 'true' 'REQ:  CF010A_104' '' } %GIDa_dabacd69_5cbb_48f9_a954_e6fb8f70c2fe"
  MotTqCmdOvrl : Outport  Port=2
  AssiCmdBasSca : Outport  RequirementInfo="{'linktype_rmi_doors' '0000c6e3 (/E-STEER Core/SubSystem Specifications/Customer Functions - EA4/GM/CF010A GM Torque Arbitrator)' '#CF010A_88' 'true' 'REQ:  CF010A_88' '' ; 'linktype_rmi_doors' '0000c6e3 (/E-STEER Core/SubSystem Specifications/Customer Functions - EA4/GM/CF010A GM Torque Arbitrator)' '#CF010A_106' 'true' 'REQ:  CF010A_106' '' } %GIDa_f97a111a_adde_4eaa_ad70_0c2b430c7a74"  Port=3
  RtnCmdSca : Outport  RequirementInfo="{'linktype_rmi_doors' '0000c6e3 (/E-STEER Core/SubSystem Specifications/Customer Functions - EA4/GM/CF010A GM Torque Arbitrator)' '#CF010A_106' 'true' 'REQ:  CF010A_106' '' ; 'linktype_rmi_doors' '0000c6e3 (/E-STEER Core/SubSystem Specifications/Customer Functions - EA4/GM/CF010A GM Torque Arbitrator)' '#CF010A_89' 'true' 'REQ:  CF010A_89' '' } %GIDa_d5f27bf1_8238_4dd9_afbe_d53788edb79d"  Port=4
  LkaTqCmdCdnd : Outport  RequirementInfo="{'linktype_rmi_doors' '0000c6e3 (/E-STEER Core/SubSystem Specifications/Customer Functions - EA4/GM/CF010A GM Torque Arbitrator)' '#CF010A_78' 'true' 'REQ:  CF010A_78' '' } %GIDa_7c0c403a_11b9_4e70_804a_59c450c0f2e7"  Port=5
  DampgCmdSca : Outport  RequirementInfo="{'linktype_rmi_doors' '0000c6e3 (/E-STEER Core/SubSystem Specifications/Customer Functions - EA4/GM/CF010A GM Torque Arbitrator)' '#CF010A_106' 'true' 'REQ:  CF010A_106' '' ; 'linktype_rmi_doors' '0000c6e3 (/E-STEER Core/SubSystem Specifications/Customer Functions - EA4/GM/CF010A GM Torque Arbitrator)' '#CF010A_90' 'true' 'REQ:  CF010A_90' '' } %GIDa_db7d3091_662c_4698_a2ba_4c7939c1107c"  Port=6
  EscCmdArbd : Outport  RequirementInfo="{'linktype_rmi_doors' '0000c6e3 (/E-STEER Core/SubSystem Specifications/Customer Functions - EA4/GM/CF010A GM Torque Arbitrator)' '#CF010A_79' 'true' 'REQ:  CF010A_79' '' } %GIDa_3136e235_cf21_416a_8ce4_ae35381c38ef"  Port=7
  EscLimdActv : Outport  RequirementInfo="{'linktype_rmi_doors' '0000c6e3 (/E-STEER Core/SubSystem Specifications/Customer Functions - EA4/GM/CF010A GM Torque Arbitrator)' '#CF010A_102' 'true' 'REQ:  CF010A_102' '' } %GIDa_1e528597_2917_44b4_bf54_824877ee6778"  Port=8
  PullCmpCustLrngDi : Outport  RequirementInfo="{'linktype_rmi_doors' '0000c6e3 (/E-STEER Core/SubSystem Specifications/Customer Functions - EA4/GM/CF010A GM Torque Arbitrator)' '#CF010A_113' 'true' 'REQ:  CF010A_113' '' } %GIDa_b9e13e92_7017_4f32_abba_1f30a44af883"  Port=9
  wires:
  ESC logic/1(ESCTqCmd) -> Data Store Write1/1, CAN Conditioning/2(ESCTqCmd)
  Constant7/1 -> THEN1/1(In1)
  MotTqServoCmd/1 -> PosnServo_Smoothed_Ramp/1(PosnServoCmd)
  Merge2/1 -> LimDyn_f2/1  "RtnCmdSca_Uls_T_f32"
  EscCmd/1 -> ESC logic/1(EscCmd)
  Merge/1 -> Add/2  "HwTqOscCmd_MotNwtMtr_T_f32"
  Add/1 -> "LimDyn_f32 "/1  "MotTqCmdOvrl_MotNwtMtr_T_f32"
  HwOscnEna/1 -> If/1
  CAN Conditioning/1(LkaTqCmdCdnd) -> LimDyn_f5/1
  Determine Desired Value/1(DesLKATqCmd) -> Data Store Write3/1, Ramp to Value/1(DesLKATqCmd)
  HwAgServoEna/1 -> PosnServo_Smoothed_Ramp/2(HwAgServoEna), Determine Desired Value/2(HwAgServoEna)
  PosnServo_Smoothed_Ramp/2(ScaleFactor) -> [ScaleFactor]
  Ramp to Value/2(LKAInterTqCmd) -> Data Store Write2/1, CAN Conditioning/1(LKAInterTqCmd)
  LkaSt/1 -> [LkaSt], Determine Desired Value/1(LkaSt)
  Constant3/1 -> If2/1
  Constant1/1 -> If1/1
  Merge3/1 -> LimDyn_f3/1  "DampgCmdSca_Uls_T_f32"
  HwTqOscCmd/1 -> THEN2/1(In1)
  LkaTqCmd/1 -> Determine Desired Value/3(LkaTqCmd)
  CAN Conditioning/3(HwTqOvrl) -> LimDyn_f32/1
  ESC logic/2(ESCLmid) -> EscLimdActv/1
  THEN3/1(Out1) -> Merge1/1
  HwTq/1 -> PosnServo_Smoothed_Ramp/3(HwTq)
  Constant5/1 -> If3/1
  PosnServo_Smoothed_Ramp/1(PosnServoTqCmd) -> Add/1
  EscSt/1 -> [EscSt], ESC logic/2(EscSt)
  CAN Conditioning/2(EscCmdArbd) -> LimDyn_f4/1
  If/2 -> THEN1/Action
  If/1 -> THEN2/Action
  THEN2/1(Out1) -> Merge/1
  THEN1/1(Out1) -> Merge/2
  [ScaleFactor] -> THEN3/1(In1)  "ScaleFactor_Uls_T_f32"
  If1/1 -> THEN3/Action
  Constant8/1 -> THEN4/1(In1)
  If1/2 -> THEN4/Action
  Merge1/1 -> LimDyn_f1/1  "AssiCmdBasSca_Uls_T_f32"
  THEN4/1(Out1) -> Merge1/2
  THEN5/1(Out1) -> Merge2/1
  [ScaleFactor] -> THEN5/1(In1)  "ScaleFactor_Uls_T_f32"
  If2/1 -> THEN5/Action
  Constant9/1 -> THEN6/1(In1)
  If2/2 -> THEN6/Action
  THEN6/1(Out1) -> Merge2/2
  THEN7/1(Out1) -> Merge3/1
  [ScaleFactor] -> THEN7/1(In1)  "ScaleFactor_Uls_T_f32"
  If3/1 -> THEN7/Action
  Constant10/1 -> THEN8/1(In1)
  If3/2 -> THEN8/Action
  THEN8/1(Out1) -> Merge3/2
  "LimDyn_f32 "/1 -> MotTqCmdOvrl/1
  Unary Minus/1 -> "LimDyn_f32 "/2
  Constant2/1 -> "LimDyn_f32 "/3, Unary Minus/1
  Constant4/1 -> LimDyn_f32/3, Unary Minus1/1
  Unary Minus1/1 -> LimDyn_f32/2
  LimDyn_f1/1 -> AssiCmdBasSca/1
  LimDyn_f2/1 -> RtnCmdSca/1
  LimDyn_f3/1 -> DampgCmdSca/1
  Constant6/1 -> LimDyn_f1/3
  Constant11/1 -> LimDyn_f2/3
  Constant12/1 -> LimDyn_f3/3
  Constant13/1 -> LimDyn_f1/2
  Constant14/1 -> LimDyn_f2/2
  Constant15/1 -> LimDyn_f3/2
  LimDyn_f32/1 -> HwTqOvrl/1
  Constant16/1 -> Unary Minus2/1, LimDyn_f4/3
  Unary Minus2/1 -> LimDyn_f4/2
  LimDyn_f4/1 -> EscCmdArbd/1
  Constant17/1 -> LimDyn_f5/3, Unary Minus3/1
  Unary Minus3/1 -> LimDyn_f5/2
  LimDyn_f5/1 -> LkaTqCmdCdnd/1
  VehSpdMaxSecur/1 -> Ramp to Value/2(VehSpdMaxSecur)
  [EscSt] -> CAN Conditioning/3(ESCSt)
  [LkaSt] -> Pull Compensation Learning Trigger/2(LkaSt)
  ESC logic/3(ESCActv) -> Pull Compensation Learning Trigger/1(ESCActv)
  Pull Compensation Learning Trigger/1(PullCmpCustLrngDi) -> PullCmpCustLrngDi/1
  Ramp to Value/1(OutpTqOvrlCmd) -> Data Store Write4/1, Add/3
